simulink model "target_driver_2022_Ctrl_v_2_4_landing_2017a"  (R2017a)
settings: Solver=FixedStepDiscrete  StartTime=0.0  StopTime=13  FixedStep=0.0001  RelTol=1e-3  EnableMultiTasking=on
values from neighbouring files (symbols this model uses):
  a2_lb = -0.25    [target_driver_setup_2022_Ctrl_V_2_4.m]    (also in target_driver_setup_2022_Ctrl_V_2_4_christian.m)
  a2_openloop = -0    (= 0)    [target_driver_setup_2022_Ctrl_V_2_4.m]    (also in target_driver_setup_2022_Ctrl_V_2_4_christian.m)
  a2_ub = 0.25    [target_driver_setup_2022_Ctrl_V_2_4.m]    (also in target_driver_setup_2022_Ctrl_V_2_4_christian.m)
  adaptive_flag = 0    [target_driver_setup_2022_Ctrl_V_2_4.m]    (also in target_driver_setup_2022_Ctrl_V_2_4_christian.m)
  adaptive_gain = [gamma_adaptive, adaptive_roll_limit, adaptive_pitch_limit, adaptive_yaw_limit, c_2_adaptive, gamma_lateral_adaptive, adaptive_x_limit, adaptive_y_limit, adaptive_z_limit, c_1_adaptive]    [target_driver_setup_2022_Ctrl_V_2_4.m]    (also in target_driver_setup_2022_Ctrl_V_2_4_christian.m)
  adaptive_lateral_flag = 0    [target_driver_setup_2022_Ctrl_V_2_4.m]    (also in target_driver_setup_2022_Ctrl_V_2_4_christian.m)
  adaptive_pitch_init = 0    [target_driver_setup_2022_Ctrl_V_2_4.m]    (also in target_driver_setup_2022_Ctrl_V_2_4_christian.m)
  adaptive_pitch_limit = 0.1/(scale^2)    (= 1e-07)    [target_driver_setup_2022_Ctrl_V_2_4.m]    (also in target_driver_setup_2022_Ctrl_V_2_4_christian.m)
  adaptive_pitch_limit_low = -adaptive_pitch_limit    (= -1e-07)    [target_driver_setup_2022_Ctrl_V_2_4.m]    (also in target_driver_setup_2022_Ctrl_V_2_4_christian.m)
  adaptive_roll_init = 0    [target_driver_setup_2022_Ctrl_V_2_4.m]    (also in target_driver_setup_2022_Ctrl_V_2_4_christian.m)
  adaptive_roll_limit = 0.3/(scale^2)    (= 3e-07)    [target_driver_setup_2022_Ctrl_V_2_4.m]    (also in target_driver_setup_2022_Ctrl_V_2_4_christian.m)
  adaptive_roll_limit_low = -adaptive_roll_limit    (= -3e-07)    [target_driver_setup_2022_Ctrl_V_2_4.m]    (also in target_driver_setup_2022_Ctrl_V_2_4_christian.m)
  adaptive_x_init = 0    [target_driver_setup_2022_Ctrl_V_2_4.m]    (also in target_driver_setup_2022_Ctrl_V_2_4_christian.m)
  adaptive_x_limit = 0.15/(scale)    (= 0.00015)    [target_driver_setup_2022_Ctrl_V_2_4.m]    (also in target_driver_setup_2022_Ctrl_V_2_4_christian.m)
  adaptive_x_limit_low = -adaptive_x_limit    (= -0.00015)    [target_driver_setup_2022_Ctrl_V_2_4.m]    (also in target_driver_setup_2022_Ctrl_V_2_4_christian.m)
  adaptive_y_init = 0    [target_driver_setup_2022_Ctrl_V_2_4.m]    (also in target_driver_setup_2022_Ctrl_V_2_4_christian.m)
  adaptive_y_limit = 0.15/(scale)    (= 0.00015)    [target_driver_setup_2022_Ctrl_V_2_4.m]    (also in target_driver_setup_2022_Ctrl_V_2_4_christian.m)
  adaptive_y_limit_low = -adaptive_y_limit    (= -0.00015)    [target_driver_setup_2022_Ctrl_V_2_4.m]    (also in target_driver_setup_2022_Ctrl_V_2_4_christian.m)
  adaptive_yaw_init = 0    [target_driver_setup_2022_Ctrl_V_2_4.m]    (also in target_driver_setup_2022_Ctrl_V_2_4_christian.m)
  adaptive_yaw_limit = 0.035/(scale^2)    (= 3.5e-08)    [target_driver_setup_2022_Ctrl_V_2_4.m]    (also in target_driver_setup_2022_Ctrl_V_2_4_christian.m)
  adaptive_yaw_limit_low = -adaptive_yaw_limit    (= -3.5e-08)    [target_driver_setup_2022_Ctrl_V_2_4.m]    (also in target_driver_setup_2022_Ctrl_V_2_4_christian.m)
  adaptive_z_init = 0/scale    (= 0)    [target_driver_setup_2022_Ctrl_V_2_4.m]    (also in target_driver_setup_2022_Ctrl_V_2_4_christian.m)
  adaptive_z_limit = 0.20/(scale)    (= 0.0002)    [target_driver_setup_2022_Ctrl_V_2_4.m]    (also in target_driver_setup_2022_Ctrl_V_2_4_christian.m)
  adaptive_z_limit_low = -adaptive_z_limit/1    (= -0.0002)    [target_driver_setup_2022_Ctrl_V_2_4.m]    (also in target_driver_setup_2022_Ctrl_V_2_4_christian.m)
  att_s = 500    [target_driver_setup_2022_Ctrl_V_2_4.m]    (also in target_driver_setup_2022_Ctrl_V_2_4_christian.m)
  b_1_d_desired = [1,0,0]    [target_driver_setup_2022_Ctrl_V_2_4.m]    (also in target_driver_setup_2022_Ctrl_V_2_4_christian.m)
  closedloop_flag = 1    [target_driver_setup_2022_Ctrl_V_2_4.m]    (also in target_driver_setup_2022_Ctrl_V_2_4_christian.m)
  control_gain = [k_x,k_v, k_R, k_Omega, k_z, k_vz, k_Rx]    [target_driver_setup_2022_Ctrl_V_2_4.m]    (also in target_driver_setup_2022_Ctrl_V_2_4_christian.m)
  delay = delay-vicon_sample_cycle/2    [target_driver_setup_2022_Ctrl_V_2_4.m]    (also in target_driver_setup_2022_Ctrl_V_2_4_christian.m)
  drv_amp = 160    [target_driver_setup_2022_Ctrl_V_2_4.m]    (also in target_driver_setup_2022_Ctrl_V_2_4_christian.m)
  drv_bias = max_drv_bias    (= 300)    [target_driver_setup_2022_Ctrl_V_2_4.m]    (also in target_driver_setup_2022_Ctrl_V_2_4_christian.m)
  drv_pitch_left = 0    [target_driver_setup_2022_Ctrl_V_2_4.m]    (also in target_driver_setup_2022_Ctrl_V_2_4_christian.m)
  drv_pitch_right = 0    [target_driver_setup_2022_Ctrl_V_2_4.m]    (also in target_driver_setup_2022_Ctrl_V_2_4_christian.m)
  drv_roll = -2    [target_driver_setup_2022_Ctrl_V_2_4.m]    (also in target_driver_setup_2022_Ctrl_V_2_4_christian.m = 0)
  f_fin = f    (= 155)    [target_driver_setup_2022_Ctrl_V_2_4.m]    (also in target_driver_setup_2022_Ctrl_V_2_4_christian.m)
  f_int = f    (= 155)    [target_driver_setup_2022_Ctrl_V_2_4.m]    (also in target_driver_setup_2022_Ctrl_V_2_4_christian.m)
  g = 9.8    [target_driver_setup_2022_Ctrl_V_2_4.m]    (also in target_driver_setup_2022_Ctrl_V_2_4_christian.m)
  I_moment_vec = [Ixx, Iyy, Izz]    [target_driver_setup_2022_Ctrl_V_2_4.m]    (also in target_driver_setup_2022_Ctrl_V_2_4_christian.m)
  landing_flag = 0    [target_driver_setup_2022_Ctrl_V_2_4.m]    (also in target_driver_setup_2022_Ctrl_V_2_4_christian.m)
  landing_parameter = [start_delay+T,transition_rate, rising_time, falling_time, landing_rising_time, landing_z_decrease, landing_y_decrease, landing_x_decrease]    [target_driver_setup_2022_Ctrl_V_2_4.m]    (also in target_driver_setup_2022_Ctrl_V_2_4_christian.m = [start_delay+T, transition_rate, rising_time, falling_time, )
  low_bound = -8    [target_driver_setup_2022_Ctrl_V_2_4.m]    (also in target_driver_setup_2022_Ctrl_V_2_4_christian.m = -10)
  low_bound_eR = -0.8    [target_driver_setup_2022_Ctrl_V_2_4.m]    (also in target_driver_setup_2022_Ctrl_V_2_4_christian.m)
  low_bound_vx = -0.5    [target_driver_setup_2022_Ctrl_V_2_4.m]    (also in target_driver_setup_2022_Ctrl_V_2_4_christian.m)
  low_bound_vy = -0.5    [target_driver_setup_2022_Ctrl_V_2_4.m]    (also in target_driver_setup_2022_Ctrl_V_2_4_christian.m)
  low_bound_vz = -0.5    [target_driver_setup_2022_Ctrl_V_2_4.m]    (also in target_driver_setup_2022_Ctrl_V_2_4_christian.m)
  low_bound_x = -0.06    [target_driver_setup_2022_Ctrl_V_2_4.m]    (also in target_driver_setup_2022_Ctrl_V_2_4_christian.m)
  low_bound_y = -0.06    [target_driver_setup_2022_Ctrl_V_2_4.m]    (also in target_driver_setup_2022_Ctrl_V_2_4_christian.m)
  low_bound_z = -0.04    [target_driver_setup_2022_Ctrl_V_2_4.m]    (also in target_driver_setup_2022_Ctrl_V_2_4_christian.m)
  m = m+payload    (= 0.000124)    [target_driver_setup_2022_Ctrl_V_2_4.m]    (also in target_driver_setup_2022_Ctrl_V_2_4_christian.m = 0.000119)
  params_vec = [params_opt.delta_1, params_opt.delta_2, params_opt.delta_3, params_opt.gamma_1, params_opt.gamma_2, params_opt.gamma_3, params_opt.eta, params_opt.nu, params_opt.mu]'    [target_driver_setup_2022_Ctrl_V_2_4.m]    (also in target_driver_setup_2022_Ctrl_V_2_4_christian.m)
  phase = 0    [target_driver_setup_2022_Ctrl_V_2_4.m]    (also in target_driver_setup_2022_Ctrl_V_2_4_christian.m)
  r_desired = [default_x, default_y,z_desired]    [target_driver_setup_2022_Ctrl_V_2_4.m]    (also in target_driver_setup_2022_Ctrl_V_2_4_christian.m)
  roll_offset_angle = 0    [target_driver_setup_2022_Ctrl_V_2_4.m]    (also in target_driver_setup_2022_Ctrl_V_2_4_christian.m)
  running_time = start_delay+total_T    (= 8.5)    [target_driver_setup_2022_Ctrl_V_2_4.m]    (also in target_driver_setup_2022_Ctrl_V_2_4_christian.m = 8.4)
  running_time_control = start_delay_control+total_T+0.0    (= 8.6)    [target_driver_setup_2022_Ctrl_V_2_4.m]    (also in target_driver_setup_2022_Ctrl_V_2_4_christian.m = 8.5)
  start_delay = 2.0    (= 2)    [target_driver_setup_2022_Ctrl_V_2_4.m]    (also in target_driver_setup_2022_Ctrl_V_2_4_christian.m)
  start_delay_control = start_delay + ramp_delay    (= 2.1)    [target_driver_setup_2022_Ctrl_V_2_4.m]    (also in target_driver_setup_2022_Ctrl_V_2_4_christian.m)
  T = 0.5    [target_driver_setup_2022_Ctrl_V_2_4.m]    (also in target_driver_setup_2022_Ctrl_V_2_4_christian.m = 0.4)
  task_flag = 0    [target_driver_setup_2022_Ctrl_V_2_4.m]    (also in target_driver_setup_2022_Ctrl_V_2_4_christian.m)
  task_parameter = [radius_ref, frequency_ref, radius_ratio, lissajous_ratio, lissajous_delta, lissajous_amplitude_ratio,z_radius_ratio]    [target_driver_setup_2022_Ctrl_V_2_4.m]    (also in target_driver_setup_2022_Ctrl_V_2_4_christian.m)
  upp_bound = 8    [target_driver_setup_2022_Ctrl_V_2_4.m]    (also in target_driver_setup_2022_Ctrl_V_2_4_christian.m = 10)
  upp_bound_eR = 0.8    [target_driver_setup_2022_Ctrl_V_2_4.m]    (also in target_driver_setup_2022_Ctrl_V_2_4_christian.m)
  upp_bound_vx = 0.5    [target_driver_setup_2022_Ctrl_V_2_4.m]    (also in target_driver_setup_2022_Ctrl_V_2_4_christian.m)
  upp_bound_vy = 0.5    [target_driver_setup_2022_Ctrl_V_2_4.m]    (also in target_driver_setup_2022_Ctrl_V_2_4_christian.m)
  upp_bound_vz = 0.5    [target_driver_setup_2022_Ctrl_V_2_4.m]    (also in target_driver_setup_2022_Ctrl_V_2_4_christian.m)
  upp_bound_x = 0.06    [target_driver_setup_2022_Ctrl_V_2_4.m]    (also in target_driver_setup_2022_Ctrl_V_2_4_christian.m)
  upp_bound_y = 0.06    [target_driver_setup_2022_Ctrl_V_2_4.m]    (also in target_driver_setup_2022_Ctrl_V_2_4_christian.m)
  upp_bound_z = 0.04    [target_driver_setup_2022_Ctrl_V_2_4.m]    (also in target_driver_setup_2022_Ctrl_V_2_4_christian.m)
undefined symbols (not defined in the file or in its folder): A, Com1, DiscIntNeverNeededParam, left_mapping, left_mapping_F_to_Phi, lp_den, lp_num, none, right_mapping, right_mapping_F_to_Phi, vlp_den, vlp_num
libraries: simulink x25, xpcnilib x2, xpcseriallib x2, xpcutilitieslib x1
(part 1 of 4)
settings Model: ExtModeArmWhenConnect=off  Creator=DEAS IT  LastModifiedBy=Wyss User
settings SolverCC: EnableConcurrentExecution=on
settings DataIOCC: LimitDataPoints=on  MaxDataPoints=1000000000  SaveFormat=Array
settings OptimizationCC: BlockReduction=off  BooleanDataType=off  OptimizeBlockIOStorage=off  BufferReuse=off  GlobalBufferReuse=off  ExpressionFolding=off  ExpressionDepthLimit=2147483647  LocalBlockOutputs=off  InitFltsAndDblsToZero=on  OptimizeDataStoreBuffers=off  BusAssignmentInplaceUpdate=off
settings DebuggingCC: SaveWithParameterizedLinksMsg=none  UnderspecifiedInitializationDetection=Classic  MergeDetectMultiDrivingBlocksExec=none  MultiTaskDSMMsg=warning  MultiTaskCondExecSysMsg=none  FcnCallInpInsideContextMsg=warning  StateNameClashWarn=warning  SFUnexpectedBacktrackingDiag=warning  SFNoUnconditionalDefaultTransitionDiag=warning  SFExecutionAtInitializationDiag=none
settings HardwareCC: ProdBitPerPointer=32  ProdBitPerSizeT=32  ProdBitPerPtrDiffT=32  ProdLargestAtomicFloat=None  ProdWordSize=32  ProdLongLongMode=on  ProdHWDeviceType=Generic->32-bit x86 compatible  TargetHWDeviceType=32-bit Generic
settings ModelReferenceCC: PropagateSignalLabelsOutOfModel=off
settings RTWCC: SystemTargetFile=slrt.tlc  TemplateMakefile=slrt_default_tmf  Description=Simulink Real-Time  RTWCompilerOptimization=on
settings SimulinkRealTimeCC: TargetFcnLib=ansi_tfl_tmw.mat  RL32LogBufSizeModifier=10000000  xPCConcurrentTasks=on
settings ConfigComp: CovMetricSettings=dw  CovHtmlReporting=on  CovSaveCumulativeToWorkspaceVar=on  CovSaveSingleToWorkspaceVar=on  CovExternalEMLEnable=off

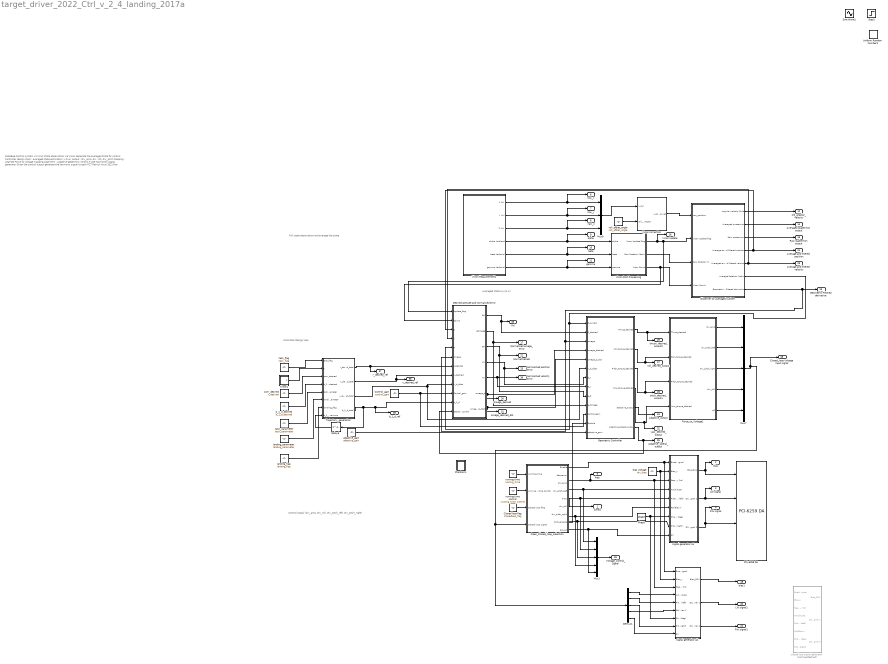
== system target_driver_2022_Ctrl_v_2_4_landing_2017a ==
  note: RoboBee Control system v2.1
      | Full state observation via Vicon
      | Generate the averaged state for control
      | Controller design
      | input : averaged state estimate (r,v,R,w)
      | output : drv_amp, drv_roll, drv_pitch
      | Mapping : Learned Force to voltage mapping
      | Algorithm : Adaptive geoemtric control T.Lee
      | Harmonitc signal generator
      | Given the control output generate the harmonic signal to each PZT
      |
      | Patrick Hyun 2021 Mar
  note: Controller Design loop
  note: Averaged state
      | (p,v,R,w)
  note: Full state observation and average the state
  note: Control signal
      | (drv_amp, drv_roll, drv_pitch_left, drv_pitch_right)
  Closed loop flag : Constant  Value=closedloop_flag
  Control_gain : Constant  Value=control_gain  SampleTime=-1
  Delay6 : Delay  DelayLength=1  InitialCondition=0
  Demux1 : Demux  Outputs=5
  Desired attitude and normalized error : Subsystem
  Force_to_Voltage1 : Subsystem
  Geometric Controller : Subsystem
  Mux1 : Mux  Inputs=5
  Mux7 : Mux  Inputs=5
  Mux9 : Mux  Inputs=3
  Observer for averaged system : Subsystem
  Open_Closed_loop_selection : Subsystem
  PCI-6259 DA : xpcnilib/D//A/M Series/PCI-6259 DA  channel=[1:4]  range=[10,5, 10, 10]  reset=[1 1 1 1]  initValue=[0 0 0 0]  sampletime=-1  slot=-1
      settings: SourceProductName=Simulink Real-Time  SourceProductBaseCode=XP
  Phantom1 : Subsystem
  Phase : Constant  Value=phase
  Trajectory_generation : MATLAB Function  TreatAsAtomicUnit=on
  Vicon Measurements : Subsystem
  Vicon Post Processing : Subsystem
  Vicon correction : MATLAB Function  TreatAsAtomicUnit=on
  adaptive_gain : Constant  Value=adaptive_gain  SampleTime=-1
  b_1_d_desired : Constant  Value=b_1_d_desired  SampleTime=-1
  bias voltage : Constant  Value=drv_bias
  closed loop signal generator : Subsystem  Commented=on
  com_desired : Constant  Value=r_desired  SampleTime=-1
  landing_flag : Constant  Value=landing_flag  SampleTime=-1
  landing_parameter : Constant  Value=landing_parameter  SampleTime=-1
  roll_offset_angle : Constant  Value=roll_offset_angle  SampleTime=-1
  running time : Constant  Value=running_time  SampleTime=-1
  running time control : Constant  Value=running_time_control  SampleTime=-1
  signal generator a1 : Subsystem
  signal generator a2 : Subsystem
  task_flag : Constant  Value=task_flag  SampleTime=-1
  task_parameter : Constant  Value=task_parameter  SampleTime=-1
  timer1 : Subsystem
  time1 : Outport
  bias : Outport  Port=2
  LW signal : Outport  Port=3
  RW signal : Outport  Port=4
  freq : Outport  Port=5
  raw_x : Outport  Port=6
  raw_y : Outport  Port=7
  raw_z : Outport  Port=8
  alpha : Outport  Port=9
  beta : Outport  Port=10
  gamma : Outport  Port=11
  "old_angular_velocity " : Outport  Port=12
  Geometric Filtered derivative : Outport  Port=13
  Averaged quaternion output : Outport  Port=14
  "Raw quaternion output " : Outport  Port=15
  Vicon Update : Outport  Port=16
  Normalized omega_error : Outport  Port=17
  Closed_loop Voltage input signal : Outport  Port=18
  bias1 : Outport  Port=19
  LW signal1 : Outport  Port=20
  RW signal1 : Outport  Port=21
  Normalized eR : Outport  Port=22
  Average and filtered velocity : Outport  Port=23
  "Average and filtered position " : Outport  Port=24
  Normalized position error : Outport  Port=25
  Voltage_control_Signal : Outport  Port=26
  roll_desired_output : Outport  Port=27
  pitch_desired_output1 : Outport  Port=28
  thrust_desired_output2 : Outport  Port=29
  omega_desired : Outport  Port=30
  omega_desired_dot : Outport  Port=31
  "yaw_desired_output " : Outport  Port=32
  Rd : Outport  Port=33
  Adaptive_output : Outport  Port=34
  Adaptive_lateral_output : Outport  Port=35
  Normalized velocity error : Outport  Port=36
  r_desired_ref : Outport  Port=37
  v_desired_ref : Outport  Port=38
  b_1_d_ref : Outport  Port=39
  Sine Wave1 : Sin  IOType=siggen  SampleTime=0
  Step1 : Step  IOType=siggen  SampleTime=0
  Uniform Random Number1 : UniformRandomNumber  IOType=siggen  SampleTime=0
  wires:
  signal generator a1/1(Bias_D2A) -> PCI-6259 DA/1, bias/1
  signal generator a1/2(D2A DriveSignal 1) -> LW signal/1, PCI-6259 DA/2
  signal generator a1/3(D2A DriveSignal 2) -> RW signal/1, PCI-6259 DA/3
  bias voltage/1 -> signal generator a2/2(Bias_v), signal generator a1/2(Bias_v)
  Phase/1 -> signal generator a2/7(Phase (deg)), signal generator a1/7(Phase (deg))
  Vicon Measurements/2(Y (m)) -> raw_y/1, Mux9/2
  Vicon Measurements/3(Z (m)) -> Mux9/3, raw_z/1
  Vicon Measurements/6(gamma (radians)) -> gamma/1, Vicon Post Processing/3(gamma)
  Vicon Measurements/5(beta (radians)) -> Vicon Post Processing/2(beta), beta/1
  Vicon Measurements/1(X (m)) -> raw_x/1, Mux9/1
  Vicon Measurements/4(alpha (radians)) -> Vicon Post Processing/1(alpha), alpha/1
  Mux7/1 -> Closed_loop Voltage input signal/1, Demux1/1, Open_Closed_loop_selection/4(Closed loop signal)
  signal generator a2/1(Bias_D2A) -> bias1/1
  signal generator a2/2(D2A DriveSignal 1) -> LW signal1/1
  signal generator a2/3(D2A DriveSignal 2) -> RW signal1/1
  Vicon Post Processing/1("Vicon Update Flag ") -> Vicon Update/1, Desired attitude and normalized error/1(Update_flag), Observer for averaged system/2(Vicon Update flag)
  Vicon Post Processing/2(Raw Rotation Matrix) -> Observer for averaged system/3("Raw Rotation M ")
  Vicon Post Processing/3("Vicon Count ") -> Desired attitude and normalized error/2(Count), Observer for averaged system/4(Vicon Count)
  Observer for averaged system/1("Angular velocity Euler ") -> "old_angular_velocity "/1
  Observer for averaged system/2(Averaged quaternion) -> Averaged quaternion output/1
  Observer for averaged system/3(Raw quaternion) -> "Raw quaternion output "/1
  Observer for averaged system/6(Average Rotation Matrix) -> Desired attitude and normalized error/5(R), Geometric Controller/1(R_current)
  Observer for averaged system/5(Averaged and filtered velocity) -> Average and filtered velocity/1, Desired attitude and normalized error/4(v)
  Observer for averaged system/4("Average and filtered position ") -> Desired attitude and normalized error/3(p), "Average and filtered position "/1
  Open_Closed_loop_selection/2(frequency) -> signal generator a2/3(frequency (hz)), signal generator a1/3(frequency (hz)), freq/1
  running time/1 -> Open_Closed_loop_selection/1(runnting time)
  running time control/1 -> Open_Closed_loop_selection/2("running time control ")
  Closed loop flag/1 -> Open_Closed_loop_selection/3(Closed loop flag)
  Open_Closed_loop_selection/3(drv_amp) -> signal generator a1/4(Amplitude), Mux1/1
  Open_Closed_loop_selection/4("drv_pitch_left ") -> signal generator a1/5(PitchBias V (left)), Mux1/2
  Open_Closed_loop_selection/5(time) -> time1/1
  Open_Closed_loop_selection/6("drv_roll ") -> signal generator a1/6(RollBias V), Mux1/4
  Open_Closed_loop_selection/7("drv_pitch_right ") -> signal generator a1/8(PitchBias V (right)), Mux1/3
  Demux1/1 -> signal generator a2/4(Amplitude)
  Demux1/2 -> signal generator a2/5(PitchBias V (left))
  Demux1/3 -> signal generator a2/8(PitchBias V (right))
  Demux1/4 -> signal generator a2/6(RollBias V)
  Mux1/1 -> Voltage_control_Signal/1
  Geometric Controller/3(Pitch_torque_desired) -> Force_to_Voltage1/3(Pitch_torque_desired), pitch_desired_output1/1
  Geometric Controller/1(Thrust_desired) -> thrust_desired_output2/1, Force_to_Voltage1/1("Thrust_desired ")
  Geometric Controller/2(roll_torque_desired) -> roll_desired_output/1, Force_to_Voltage1/2(Roll_torque_desired)
  Open_Closed_loop_selection/1("Enable ") -> signal generator a2/1(EnableSignal), signal generator a1/1(EnableSignal)
  Trajectory_generation/3(x_d_ddot_total) -> Desired attitude and normalized error/9(x_d_ddot), Geometric Controller/6(x_d_ddot)
  Control_gain/1 -> Geometric Controller/11(control_gain), Desired attitude and normalized error/10(Control_gain)
  Trajectory_generation/2(v_desired_total) -> v_desired_ref/1, Desired attitude and normalized error/8(v_desired)
  Desired attitude and normalized error/2(eOmega) -> Geometric Controller/10(e_Omega), Normalized omega_error/1
  Desired attitude and normalized error/3(eR) -> Geometric Controller/9(e_R), Normalized eR/1
  Desired attitude and normalized error/4(ex) -> Geometric Controller/7(e_x), Normalized position error/1
  Desired attitude and normalized error/1(Rd) -> Geometric Controller/2(R_desired), Rd/1
  Observer for averaged system/7(Geometric filtered derivative) -> Geometric Controller/3(omega), Desired attitude and normalized error/6(omega), Geometric Filtered derivative/1
  Desired attitude and normalized error/6(omega_d) -> Geometric Controller/4(omega_desired), omega_desired/1
  Desired attitude and normalized error/7(omega_d_ddot) -> Geometric Controller/5(omega_d_dot), omega_desired_dot/1
  Desired attitude and normalized error/5(ev) -> Normalized velocity error/1, Geometric Controller/8(e_v)
  Open_Closed_loop_selection/9(a2_out) -> Mux1/5, signal generator a1/9(a2)
  Open_Closed_loop_selection/8(Cntrl_enable) -> Geometric Controller/12(Enable)
  Geometric Controller/4(Yaw_torque_desired) -> "yaw_desired_output "/1, Force_to_Voltage1/4(Yaw_torque_desired)
  Force_to_Voltage1/1(drv_amp) -> Mux7/1
  Force_to_Voltage1/2(drv_pitch_left) -> Mux7/2
  Force_to_Voltage1/3(drv_pitch_right) -> Mux7/3
  Force_to_Voltage1/4(drv_roll) -> Mux7/4
  Force_to_Voltage1/5(a2) -> Mux7/5
  Demux1/5 -> signal generator a2/9(a2)
  Trajectory_generation/4(b_1_d_total) -> Delay6/1, b_1_d_ref/1, Desired attitude and normalized error/11(b_1_d)
  adaptive_gain/1 -> Geometric Controller/13(adaptive_gain)
  Geometric Controller/5(adaptive_output) -> Adaptive_output/1
  Geometric Controller/6(adaptive_lateral_output) -> Desired attitude and normalized error/12(adaptive_lateral_control), Adaptive_lateral_output/1
  Mux9/1 -> Vicon correction/1(x_cur)
  roll_offset_angle/1 -> Vicon correction/2(roll_offset_angle)
  Vicon correction/1(x_corrected_vec) -> Observer for averaged system/1("raw_position ")
  com_desired/1 -> Trajectory_generation/3(com_desired)
  Trajectory_generation/1(r_desired_total) -> r_desired_ref/1, Desired attitude and normalized error/7(r_desired)
  timer1/1(time) -> Trajectory_generation/2(t)
  task_flag/1 -> Trajectory_generation/1(task_flag)
  b_1_d_desired/1 -> Trajectory_generation/4(b_1_d_desired)
  task_parameter/1 -> Trajectory_generation/5(task_parameter)
  landing_parameter/1 -> Trajectory_generation/6(landing_parameter)
  landing_flag/1 -> Trajectory_generation/7(landing_flag)
  Delay6/1 -> Trajectory_generation/8(b_1_d_previous)

== system target_driver_2022_Ctrl_v_2_4_landing_2017a/Desired attitude and normalized error ==
  Update_flag : Inport
  Count : Inport  Port=2
  p : Inport  Port=3
  v : Inport  Port=4
  R : Inport  Port=5
  omega : Inport  Port=6
  r_desired : Inport  Port=7
  v_desired : Inport  Port=8
  x_d_ddot : Inport  Port=9
  Control_gain : Inport  Port=10
  b_1_d : Inport  Port=11
  adaptive_lateral_control : Inport  Port=12
  Delay6 : Delay  DelayLength=1  InitialCondition=0
  "Desired_Attitude " : MATLAB Function  TreatAsAtomicUnit=on
  Geometric derivative for Rd in SO(3) : Subsystem
  m : Constant  Value=m
  m1 : Constant  Value=g
  saturated normalized error observation : Subsystem
  Rd : Outport
  eOmega : Outport  Port=2
  eR : Outport  Port=3
  ex : Outport  Port=4
  ev : Outport  Port=5
  omega_d : Outport  Port=6
  omega_d_ddot : Outport  Port=7
  wires:
  r_desired/1 -> saturated normalized error observation/7(r_desired)
  x_d_ddot/1 -> "Desired_Attitude "/5(x_d_ddot)
  saturated normalized error observation/3("Normalized position error ") -> ex/1, "Desired_Attitude "/3(e_x)
  Delay6/1 -> Geometric derivative for Rd in SO(3)/1(Previous Averaged Rotation M), "Desired_Attitude "/2(R_d_prev)
  omega/1 -> saturated normalized error observation/4(omega)
  "Desired_Attitude "/1(R_d_vec) -> saturated normalized error observation/6(R_desired), Delay6/1, Rd/1, Geometric derivative for Rd in SO(3)/3(Current Averaged Rotation M)
  saturated normalized error observation/2(Normalized eR) -> eR/1
  Count/1 -> Geometric derivative for Rd in SO(3)/2(Vicon Count)
  Update_flag/1 -> "Desired_Attitude "/10(update), Geometric derivative for Rd in SO(3)/4("Vicon Update Flag ")
  p/1 -> saturated normalized error observation/1(p)
  Control_gain/1 -> "Desired_Attitude "/7(control_gain)
  v_desired/1 -> saturated normalized error observation/8("v_desired ")
  Geometric derivative for Rd in SO(3)/2(Filtered Geometric derivative ddRd in SO(3)1) -> omega_d_ddot/1
  v/1 -> saturated normalized error observation/2(v)
  saturated normalized error observation/1("Normalized omega error ") -> eOmega/1
  saturated normalized error observation/4(Normalized velocity error) -> "Desired_Attitude "/4(e_v), ev/1
  R/1 -> "Desired_Attitude "/1(R_cur), saturated normalized error observation/3(R)
  Geometric derivative for Rd in SO(3)/1(Filtered Geometric derivative dRd in SO(3)) -> saturated normalized error observation/5("omega_desired "), omega_d/1
  m/1 -> "Desired_Attitude "/8(m)
  m1/1 -> "Desired_Attitude "/9(g)
  b_1_d/1 -> "Desired_Attitude "/6(b_1_d)
  adaptive_lateral_control/1 -> "Desired_Attitude "/11(adaptive_lateral_control)

== system target_driver_2022_Ctrl_v_2_4_landing_2017a/Force_to_Voltage1 ==
  note: Mapping from desired Thrust/Torque to Wing traj to Voltage mapping
      |
      | Patrick Hyun 2021 Apr
  "Thrust_desired " : Inport
  Roll_torque_desired : Inport  Port=2
  Pitch_torque_desired : Inport  Port=3
  Yaw_torque_desired : Inport  Port=4
  A : Constant  Commented=on  Value=A
  Desired_Force_to_Voltage : MATLAB Function  TreatAsAtomicUnit=on
  "Force to Trajectory " : MATLAB Function  Commented=on  TreatAsAtomicUnit=on
  Saturation : Saturate  UpperLimit=a2_ub  LowerLimit=a2_lb
  "Trajectory to Voltage Input " : MATLAB Function  Commented=on  TreatAsAtomicUnit=on
  left_mapping : Constant  Commented=on  Value=left_mapping
  left_mapping_F_to_Phi : Constant  Commented=on  Value=left_mapping_F_to_Phi
  params_vec : Constant  Value=params_vec
  right_mapping1 : Constant  Commented=on  Value=right_mapping
  right_mapping_F_to_Phi : Constant  Commented=on  Value=right_mapping_F_to_Phi
  drv_amp : Outport
  drv_pitch_left : Outport  Port=2
  drv_pitch_right : Outport  Port=3
  drv_roll : Outport  Port=4
  a2 : Outport  Port=5
  wires:
  left_mapping/1 -> "Trajectory to Voltage Input "/4(left_mapping)
  right_mapping1/1 -> "Trajectory to Voltage Input "/5(right_mapping)
  A/1 -> "Force to Trajectory "/6(A)
  "Force to Trajectory "/1(Phi_left_p2p_desired) -> "Trajectory to Voltage Input "/1(Phi_left_p2p_command)
  "Force to Trajectory "/2(Phi_right_p2p_desired) -> "Trajectory to Voltage Input "/2(Phi_right_p2p_command)
  "Force to Trajectory "/3(Phi_pitch_desired) -> "Trajectory to Voltage Input "/3(Phi_pitch_command)
  left_mapping_F_to_Phi/1 -> "Force to Trajectory "/4(left_mapping_F_to_Phi)
  right_mapping_F_to_Phi/1 -> "Force to Trajectory "/5(right_mapping_F_to_Phi)
  Desired_Force_to_Voltage/4(drv_pitch_right) -> drv_pitch_right/1
  Desired_Force_to_Voltage/3(drv_pitch_left) -> drv_pitch_left/1
  Desired_Force_to_Voltage/2(drv_roll) -> drv_roll/1
  Desired_Force_to_Voltage/1(drv_amp) -> drv_amp/1
  "Thrust_desired "/1 -> Desired_Force_to_Voltage/1(Thrust_desired)
  Roll_torque_desired/1 -> Desired_Force_to_Voltage/2(Roll_torque_desired)
  Pitch_torque_desired/1 -> Desired_Force_to_Voltage/3(Pitch_torque_desired)
  Yaw_torque_desired/1 -> Desired_Force_to_Voltage/4(Yaw_torque_desired)
  params_vec/1 -> Desired_Force_to_Voltage/5(params_vec)
  Desired_Force_to_Voltage/5(a2_coeff) -> Saturation/1
  Saturation/1 -> a2/1

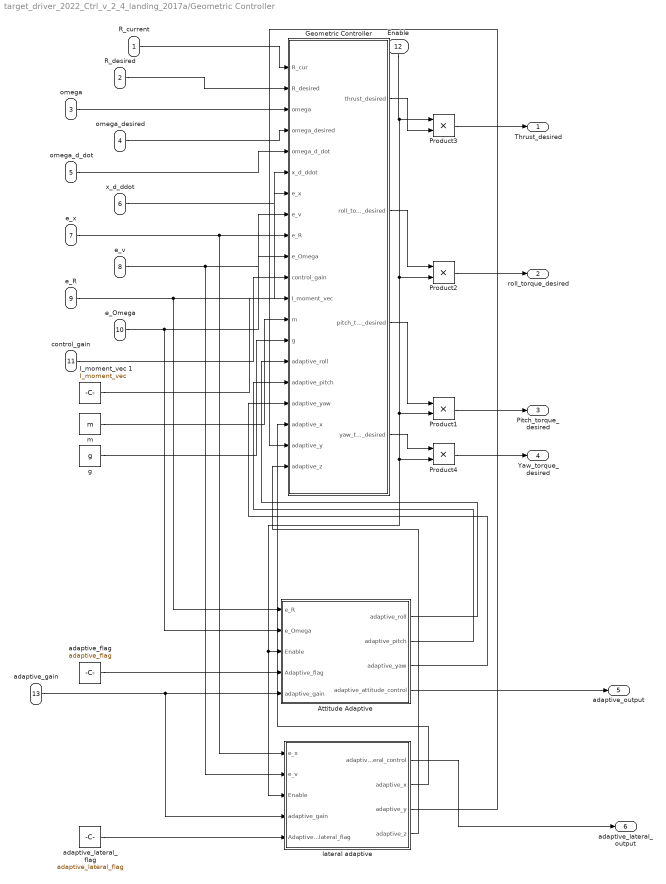
== system target_driver_2022_Ctrl_v_2_4_landing_2017a/Geometric Controller ==
  R_current : Inport
  R_desired : Inport  Port=2
  omega : Inport  Port=3
  omega_desired : Inport  Port=4
  omega_d_dot : Inport  Port=5
  x_d_ddot : Inport  Port=6
  e_x : Inport  Port=7
  e_v : Inport  Port=8
  e_R : Inport  Port=9
  e_Omega : Inport  Port=10
  control_gain : Inport  Port=11
  Enable : Inport  Port=12
  adaptive_gain : Inport  Port=13
  Attitude Adaptive : Subsystem
  Geometric Controller : MATLAB Function  TreatAsAtomicUnit=on
  I_moment_vec 1 : Constant  Value=I_moment_vec
  Product{1..4} (4 alike) : Product  RndMeth=Zero
  adaptive_flag : Constant  Value=adaptive_flag
  adaptive_lateral_flag : Constant  Value=adaptive_lateral_flag
  g : Constant  Value=g
  lateral adaptive : Subsystem
  m : Constant  Value=m
  Thrust_desired : Outport
  roll_torque_desired : Outport  Port=2
  Pitch_torque_desired : Outport  Port=3
  Yaw_torque_desired : Outport  Port=4
  adaptive_output : Outport  Port=5
  adaptive_lateral_output : Outport  Port=6
  wires:
  Product3/1 -> Thrust_desired/1
  Geometric Controller/3(pitch_torque_desired) -> Product1/1
  I_moment_vec 1/1 -> Geometric Controller/12(I_moment_vec)
  Product2/1 -> roll_torque_desired/1
  Product1/1 -> Pitch_torque_desired/1
  Geometric Controller/2(roll_torque_desired) -> Product2/1
  R_current/1 -> Geometric Controller/1(R_cur)
  Geometric Controller/1(thrust_desired) -> Product3/2
  R_desired/1 -> Geometric Controller/2(R_desired)
  omega/1 -> Geometric Controller/3(omega)
  omega_desired/1 -> Geometric Controller/4(omega_desired)
  omega_d_dot/1 -> Geometric Controller/5(omega_d_dot)
  e_R/1 -> Attitude Adaptive/1(e_R), Geometric Controller/9(e_R)
  e_Omega/1 -> Attitude Adaptive/2(e_Omega), Geometric Controller/10(e_Omega)
  control_gain/1 -> Geometric Controller/11(control_gain)
  g/1 -> Geometric Controller/14(g)
  m/1 -> Geometric Controller/13(m)
  x_d_ddot/1 -> Geometric Controller/6(x_d_ddot)
  adaptive_flag/1 -> Attitude Adaptive/4(Adaptive_flag)
  adaptive_gain/1 -> lateral adaptive/4(adaptive_gain), Attitude Adaptive/5(adaptive_gain)
  Attitude Adaptive/1(adaptive_roll) -> Geometric Controller/15(adaptive_roll)
  Attitude Adaptive/2(adaptive_pitch) -> Geometric Controller/16(adaptive_pitch)
  Attitude Adaptive/3(adaptive_yaw) -> Geometric Controller/17(adaptive_yaw)
  Attitude Adaptive/4(adaptive_attitude_control) -> adaptive_output/1
  Enable/1 -> Product4/2, Attitude Adaptive/3(Enable), lateral adaptive/3(Enable), Product1/2, Product2/2, Product3/1
  Geometric Controller/4(yaw_torque_desired) -> Product4/1
  Product4/1 -> Yaw_torque_desired/1
  e_x/1 -> Geometric Controller/7(e_x), lateral adaptive/1(e_x)
  e_v/1 -> lateral adaptive/2(e_v), Geometric Controller/8(e_v)
  adaptive_lateral_flag/1 -> lateral adaptive/5(Adaptive_lateral_flag)
  lateral adaptive/1(adaptive_lateral_control) -> adaptive_lateral_output/1
  lateral adaptive/2(adaptive_x) -> Geometric Controller/18(adaptive_x)
  lateral adaptive/3(adaptive_y) -> Geometric Controller/19(adaptive_y)
  lateral adaptive/4(adaptive_z) -> Geometric Controller/20(adaptive_z)

== system target_driver_2022_Ctrl_v_2_4_landing_2017a/Observer for averaged system ==
  note: Observer for averaged system using geoemtric average
      | Includes the Euler derivatives to compute the angular velocity (probably not used for control)
      | Includes the geometric average and the first order derivative in Riemannian metric SO(3)
      |
      | Patrick 2021 Mar
  "raw_position " : Inport
  Vicon Update flag : Inport  Port=2
  "Raw Rotation M " : Inport  Port=3
  Vicon Count : Inport  Port=4
  Attitude Observer : Subsystem
  "Euler derivative & filtered angular velocity " : Subsystem
  Position Observer : Subsystem
  Terminator : Terminator
  "Angular velocity Euler " : Outport
  Averaged quaternion : Outport  Port=2
  Raw quaternion : Outport  Port=3
  "Average and filtered position " : Outport  Port=4
  Averaged and filtered velocity : Outport  Port=5
  Average Rotation Matrix : Outport  Port=6
  Geometric filtered derivative : Outport  Port=7
  wires:
  "Raw Rotation M "/1 -> "Euler derivative & filtered angular velocity "/1("Rotation matrix "), Attitude Observer/2(Raw Rotation)
  Vicon Count/1 -> Attitude Observer/3(Vicon Count), Position Observer/3(Vicon Count)
  "raw_position "/1 -> Position Observer/1("raw_position ")
  Position Observer/1(Average and filtered position) -> "Average and filtered position "/1
  Position Observer/2(Averaged and filtered velocity) -> Averaged and filtered velocity/1
  "Euler derivative & filtered angular velocity "/1(Angular velocity_Euler) -> "Angular velocity Euler "/1
  Vicon Update flag/1 -> Attitude Observer/1(Vicon Update flag), Position Observer/2(vicon Update)
  Attitude Observer/1("Averaged quaternion ") -> Averaged quaternion/1
  Attitude Observer/2(Average Rotation Matrix) -> Average Rotation Matrix/1
  Attitude Observer/3(Raw quaternion) -> Raw quaternion/1
  Attitude Observer/4(Geometric filtered derivative) -> Geometric filtered derivative/1
  "Euler derivative & filtered angular velocity "/2(Frob_norm error) -> Terminator/1

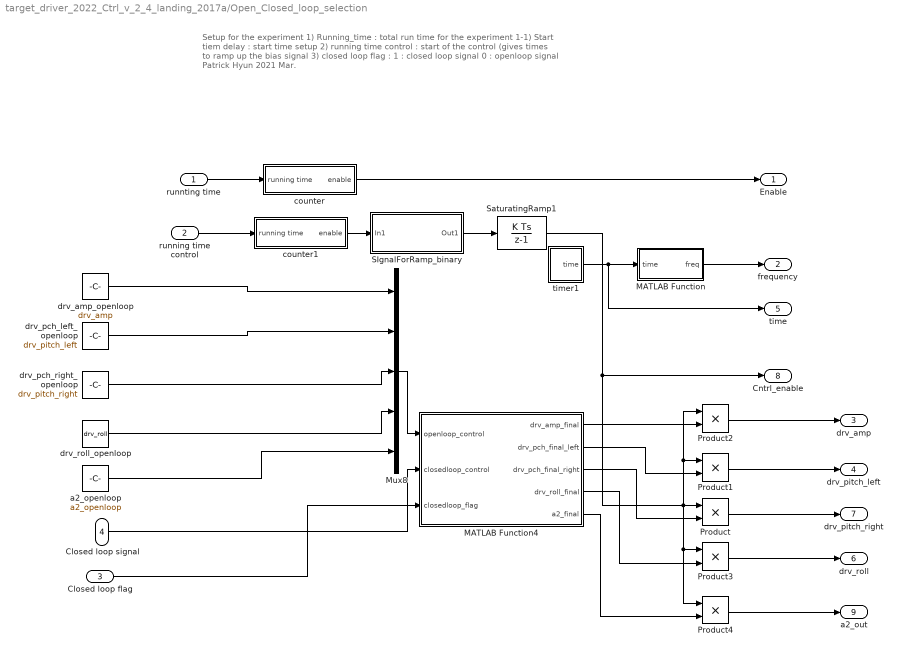
== system target_driver_2022_Ctrl_v_2_4_landing_2017a/Open_Closed_loop_selection ==
  note: Setup for the experiment
      |
      | 1) Running_time : total run time for the experiment
      | 1-1) Start tiem delay : start time setup
      | 2) running time control : start of the control (gives times to ramp up the bias signal
      | 3) closed loop flag : 1 : closed loop signal 0 : openloop signal
      |
      | Patrick Hyun 2021 Mar.
  runnting time : Inport
  "running time control " : Inport  Port=2
  Closed loop flag : Inport  Port=3
  Closed loop signal : Inport  Port=4
  MATLAB Function : MATLAB Function  TreatAsAtomicUnit=on
  MATLAB Function4 : MATLAB Function  TreatAsAtomicUnit=on
  Mux8 : Mux  Inputs=5
  Product{,1..4} (5 alike) : Product  RndMeth=Zero
  SIgnalForRamp_binary : Subsystem
  SaturatingRamp1 : DiscreteIntegrator  gainval=10  SampleTime=-1  LimitOutput=on  UpperSaturationLimit=1  LowerSaturationLimit=0  ICPrevOutput=DiscIntNeverNeededParam  ICPrevScaledInput=DiscIntNeverNeededParam
  a2_openloop : Constant  Value=a2_openloop
  counter : Subsystem
  counter1 : Subsystem
  "drv_amp_openloop " : Constant  Value=drv_amp
  drv_pch_left_openloop : Constant  Value=drv_pitch_left
  drv_pch_right_openloop : Constant  Value=drv_pitch_right
  "drv_roll_openloop " : Constant  Value=drv_roll
  timer1 : Subsystem
  "Enable " : Outport
  frequency : Outport  Port=2
  drv_amp : Outport  Port=3
  "drv_pitch_left " : Outport  Port=4
  time : Outport  Port=5
  "drv_roll " : Outport  Port=6
  "drv_pitch_right " : Outport  Port=7
  Cntrl_enable : Outport  Port=8
  a2_out : Outport  Port=9
  wires:
  runnting time/1 -> counter/1(running time)
  timer1/1(time) -> time/1, MATLAB Function/1(time)
  MATLAB Function/1(freq) -> frequency/1
  SIgnalForRamp_binary/1(Out1) -> SaturatingRamp1/1
  "drv_amp_openloop "/1 -> Mux8/1
  Product1/1 -> "drv_pitch_left "/1
  counter1/1(enable) -> SIgnalForRamp_binary/1(In1)
  "running time control "/1 -> counter1/1(running time)
  Product3/1 -> "drv_roll "/1
  SaturatingRamp1/1 -> Cntrl_enable/1, Product4/1, Product3/1, Product2/1, Product1/1, Product/1
  Closed loop flag/1 -> MATLAB Function4/3(closedloop_flag)
  MATLAB Function4/4(drv_roll_final) -> Product3/2
  Mux8/1 -> MATLAB Function4/1(openloop_control)
  MATLAB Function4/2(drv_pch_final_left) -> Product1/2
  Product2/1 -> drv_amp/1
  MATLAB Function4/1(drv_amp_final) -> Product2/2
  drv_pch_left_openloop/1 -> Mux8/2
  MATLAB Function4/3(drv_pch_final_right) -> Product/2
  Product/1 -> "drv_pitch_right "/1
  counter/1(enable) -> "Enable "/1
  Closed loop signal/1 -> MATLAB Function4/2(closedloop_control)
  "drv_roll_openloop "/1 -> Mux8/4
  drv_pch_right_openloop/1 -> Mux8/3
  Product4/1 -> a2_out/1
  MATLAB Function4/5(a2_final) -> Product4/2
  a2_openloop/1 -> Mux8/5

== system target_driver_2022_Ctrl_v_2_4_landing_2017a/Phantom1 ==
  note: high-speed camera trigger
  PCI-6259 DO1 : xpcnilib/Digital Output/M Series/PCI-6259 DO  channel=[1 2]  reset=[0 0]  initValue=[0 0]  sampletime=0.0001  slot=-1
      settings: SourceProductName=Simulink Real-Time  SourceProductBaseCode=XP
  Switch2 : Switch  Criteria=u2 > Threshold
  conv : DataTypeConversion  OutDataTypeStr=double
  pretrigger : Constant
  start at three : MATLAB Function  TreatAsAtomicUnit=on
  timer1 : Subsystem
  trigger_camera : Constant
  zero : Constant  Value=0
  wires:
  timer1/1(time) -> start at three/1(time)
  start at three/1(trigger) -> Switch2/1
  Switch2/1 -> conv/1
  zero/1 -> Switch2/3
  trigger_camera/1 -> Switch2/2
  conv/1 -> PCI-6259 DO1/2
  pretrigger/1 -> PCI-6259 DO1/1

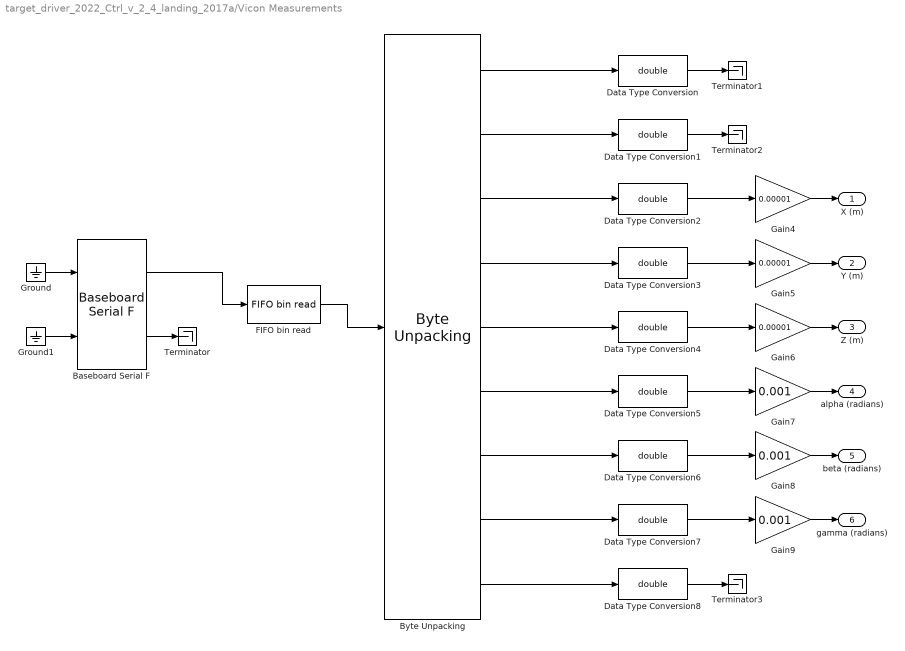
== system target_driver_2022_Ctrl_v_2_4_landing_2017a/Vicon Measurements ==
  Baseboard Serial F : xpcseriallib/Mainboard/Baseboard Serial F  group=FIFO Setup  port=1  irqnum=4  saddr1=0x3f8  saddr2=0x3e8  config=Com1/none  baud1=115200  parity1=None  ndata1=8  nstop1=1  fifomode1=16 deep  rlevel1=half full  automode1=on  xmtfifosize1=1024  xmtdatatype1=8 bit int null terminated  rcvfifosize1=1024  baud2=115200  parity2=None  ndata2=8  nstop2=1  fifomode2=16 deep  rlevel2=half full  automode2=off  xmtfifosize2=1024  xmtdatatype2=8 bit uint null terminated  rcvfifosize2=1024
      settings: SourceProductName=Simulink Real-Time  SourceProductBaseCode=XP
  "Byte Unpacking " : xpcutilitieslib/Byte Unpacking   MaskUnpackedDataTypes={'uint8','int16','int16','int16','int16','int16','int16','int16','uint8'}  MaskUnpackedDataSizes={[1] [1] [1] [1] [1] [1] [1] [1] [1]}  MaskAlignment=1
      settings: SourceProductName=Simulink Real-Time  SourceProductBaseCode=XP
  Data Type Conversion{,1..8} (9 alike) : DataTypeConversion  OutDataTypeStr=double
  "FIFO bin read " : xpcseriallib/FIFO bin read   header=[128,127,127]  lengths=[15]  hold=Hold last output if no new data  enable=off  maxsize=15  outputtype=8 bit uint null terminated  sampletime=0.0001
      settings: SourceProductName=Simulink Real-Time  SourceProductBaseCode=XP
  Gain4 : Gain  Gain=0.00001
  Gain5 : Gain  Gain=0.00001
  Gain6 : Gain  Gain=0.00001
  Gain7 : Gain  Gain=0.001
  Gain8 : Gain  Gain=0.001
  Gain9 : Gain  Gain=0.001
  Ground : Ground
  Ground1 : Ground
  Terminator{,1..3} (4 alike) : Terminator
  X (m) : Outport
  Y (m) : Outport  Port=2
  Z (m) : Outport  Port=3
  alpha (radians) : Outport  Port=4
  beta (radians) : Outport  Port=5
  gamma (radians) : Outport  Port=6
  wires:
  Baseboard Serial F/1 -> "FIFO bin read "/1
  Baseboard Serial F/2 -> Terminator/1
  Ground1/1 -> Baseboard Serial F/2
  Ground/1 -> Baseboard Serial F/1
  "Byte Unpacking "/1 -> Data Type Conversion/1
  "Byte Unpacking "/2 -> Data Type Conversion1/1
  "Byte Unpacking "/3 -> Data Type Conversion2/1
  "Byte Unpacking "/4 -> Data Type Conversion3/1
  "FIFO bin read "/1 -> "Byte Unpacking "/1
  "Byte Unpacking "/8 -> Data Type Conversion7/1
  "Byte Unpacking "/7 -> Data Type Conversion6/1
  "Byte Unpacking "/5 -> Data Type Conversion4/1
  "Byte Unpacking "/6 -> Data Type Conversion5/1
  Data Type Conversion3/1 -> Gain5/1
  Data Type Conversion4/1 -> Gain6/1
  Data Type Conversion5/1 -> Gain7/1
  Data Type Conversion6/1 -> Gain8/1
  Data Type Conversion7/1 -> Gain9/1
  "Byte Unpacking "/9 -> Data Type Conversion8/1
  Gain4/1 -> X (m)/1
  Data Type Conversion2/1 -> Gain4/1
  Gain5/1 -> Y (m)/1
  Gain6/1 -> Z (m)/1
  Gain7/1 -> alpha (radians)/1
  Gain8/1 -> beta (radians)/1
  Gain9/1 -> gamma (radians)/1
  Data Type Conversion/1 -> Terminator1/1
  Data Type Conversion1/1 -> Terminator2/1
  Data Type Conversion8/1 -> Terminator3/1

== system target_driver_2022_Ctrl_v_2_4_landing_2017a/Vicon Post Processing ==
  note: Process Vicon data
      |
      | 1) Generate Raw rotation matrix
      | 2) Flag the update of new vicon data
      | 3) Count the number of samples before new update
      |
      | By Patrick 2021 Mar
  alpha : Inport
  beta : Inport  Port=2
  gamma : Inport  Port=3
  Raw rotation matrix : Subsystem
  Vicon Validity check : Subsystem
  Vicon correction : MATLAB Function  TreatAsAtomicUnit=on
  roll_offset_angle : Constant  Value=roll_offset_angle  SampleTime=-1
  "Vicon Update Flag " : Outport
  Raw Rotation Matrix : Outport  Port=2
  "Vicon Count " : Outport  Port=3
  wires:
  Vicon Validity check/2(Vicon Count) -> "Vicon Count "/1
  beta/1 -> Raw rotation matrix/2(beta)
  gamma/1 -> Raw rotation matrix/3(gamma)
  alpha/1 -> Raw rotation matrix/1(alpha)
  Vicon Validity check/1("Vicon Update flag ") -> "Vicon Update Flag "/1
  roll_offset_angle/1 -> Vicon correction/2(roll_offset_angle)
  Raw rotation matrix/1(R) -> Vicon correction/1(R_cur)
  Vicon correction/1(Rot_corrected_vec) -> Raw Rotation Matrix/1, Vicon Validity check/1("Rotation Matrix ")

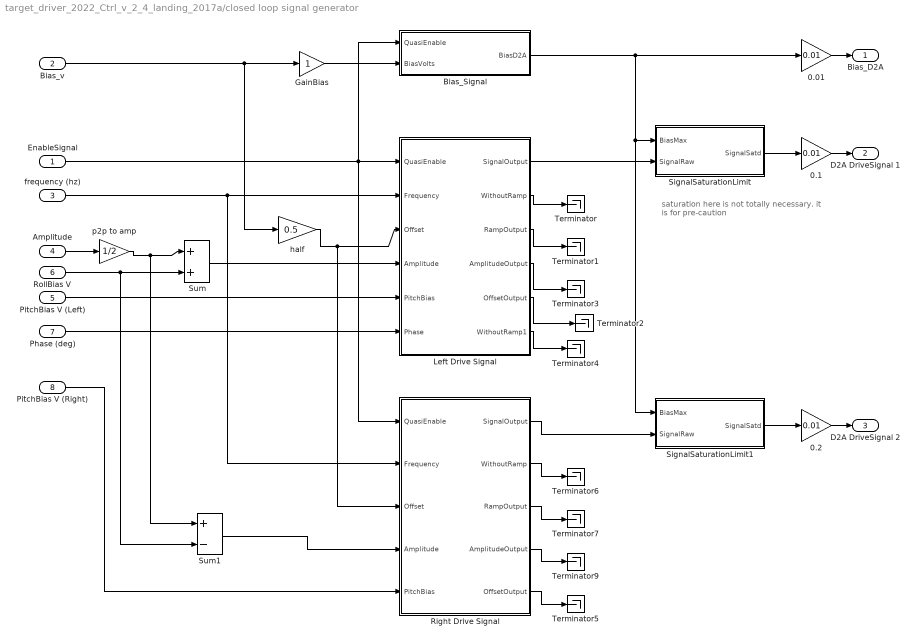
== system target_driver_2022_Ctrl_v_2_4_landing_2017a/closed loop signal generator ==
  note: saturation here is not totally necessary.
      | it is for pre-caution
  EnableSignal : Inport
  Bias_v : Inport  Port=2
  frequency (hz) : Inport  Port=3
  Amplitude : Inport  Port=4
  PitchBias V (Left) : Inport  Port=5
  RollBias V : Inport  Port=6
  Phase (deg) : Inport  Port=7
  PitchBias V (Right) : Inport  Port=8
  0.01 : Gain  Gain=0.01
  0.1 : Gain  Gain=0.01
  0.2 : Gain  Gain=0.01
  Bias_Signal : Subsystem
  GainBias : Gain
  "Left Drive Signal " : Subsystem
  Right Drive Signal : Subsystem
  SignalSaturationLimit : Subsystem
  SignalSaturationLimit1 : Subsystem
  Sum : Sum
  Sum1 : Sum  Inputs=+-
  Terminator{,1..7,9} (9 alike) : Terminator
  half : Gain  Gain=0.5
  p2p to amp : Gain  Gain=1/2
  Bias_D2A : Outport
  D2A DriveSignal 1 : Outport  Port=2
  D2A DriveSignal 2 : Outport  Port=3
  wires:
  Bias_Signal/1(BiasD2A) -> SignalSaturationLimit1/1(BiasMax), SignalSaturationLimit/1(BiasMax), 0.01/1
  half/1 -> "Left Drive Signal "/3(Offset), Right Drive Signal/3(Offset)
  Bias_v/1 -> GainBias/1, half/1
  EnableSignal/1 -> "Left Drive Signal "/1(QuasiEnable), Bias_Signal/1(QuasiEnable), Right Drive Signal/1(QuasiEnable)
  frequency (hz)/1 -> Right Drive Signal/2(Frequency), "Left Drive Signal "/2(Frequency)
  "Left Drive Signal "/2(WithoutRamp) -> Terminator/1
  "Left Drive Signal "/3(RampOutput) -> Terminator1/1
  "Left Drive Signal "/5(OffsetOutput) -> Terminator2/1
  SignalSaturationLimit/1(SignalSatd) -> 0.1/1
  GainBias/1 -> Bias_Signal/2(BiasVolts)
  Sum/1 -> "Left Drive Signal "/4(Amplitude)
  RollBias V/1 -> Sum/2, Sum1/2
  SignalSaturationLimit1/1(SignalSatd) -> 0.2/1
  Right Drive Signal/5(OffsetOutput) -> Terminator5/1
  Amplitude/1 -> p2p to amp/1
  p2p to amp/1 -> Sum/1, Sum1/1
  "Left Drive Signal "/4(AmplitudeOutput) -> Terminator3/1
  Right Drive Signal/2(WithoutRamp) -> Terminator6/1
  Right Drive Signal/3(RampOutput) -> Terminator7/1
  Right Drive Signal/4(AmplitudeOutput) -> Terminator9/1
  0.01/1 -> Bias_D2A/1
  0.1/1 -> D2A DriveSignal 1/1
  0.2/1 -> D2A DriveSignal 2/1
  Sum1/1 -> Right Drive Signal/4(Amplitude)
  Right Drive Signal/1(SignalOutput) -> SignalSaturationLimit1/2(SignalRaw)
  "Left Drive Signal "/1(SignalOutput) -> SignalSaturationLimit/2(SignalRaw)
  Phase (deg)/1 -> "Left Drive Signal "/6(Phase)
  "Left Drive Signal "/6(WithoutRamp1) -> Terminator4/1
  PitchBias V (Left)/1 -> "Left Drive Signal "/5(PitchBias)
  PitchBias V (Right)/1 -> Right Drive Signal/5(PitchBias)

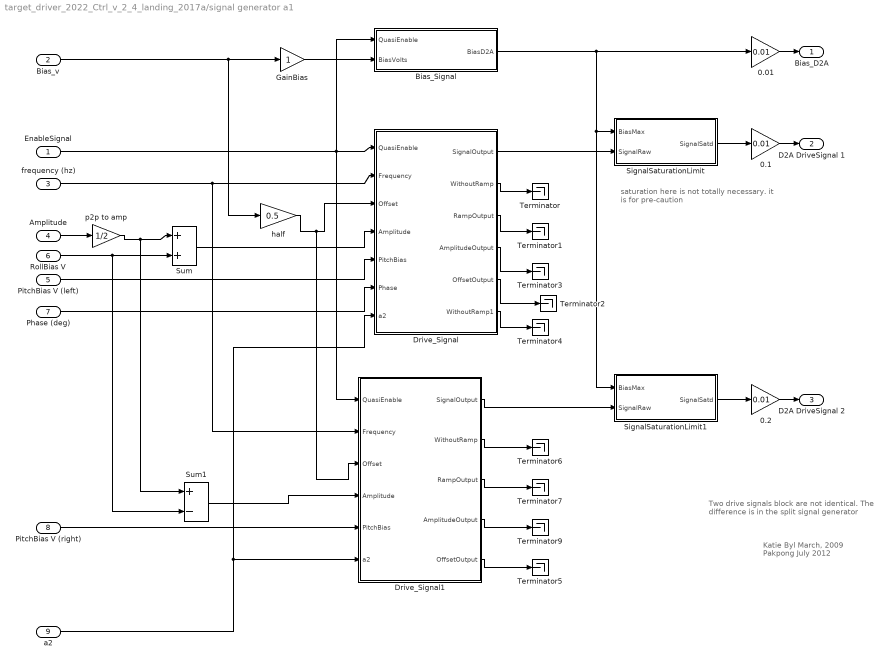
== system target_driver_2022_Ctrl_v_2_4_landing_2017a/signal generator a1 ==
  note: Katie Byl
      | March, 2009
      |
      | Pakpong
      | July 2012
  note: Two drive signals block are not identical.
      | The difference is in the split signal generator
  note: saturation here is not totally necessary.
      | it is for pre-caution
  EnableSignal : Inport
  Bias_v : Inport  Port=2
  frequency (hz) : Inport  Port=3
  Amplitude : Inport  Port=4
  PitchBias V (left) : Inport  Port=5
  RollBias V : Inport  Port=6
  Phase (deg) : Inport  Port=7
  PitchBias V (right) : Inport  Port=8
  a2 : Inport  Port=9
  0.01 : Gain  Gain=0.01
  0.1 : Gain  Gain=0.01
  0.2 : Gain  Gain=0.01
  Bias_Signal : Subsystem
  Drive_Signal : Subsystem
  Drive_Signal1 : Subsystem
  GainBias : Gain
  SignalSaturationLimit : Subsystem
  SignalSaturationLimit1 : Subsystem
  Sum : Sum
  Sum1 : Sum  Inputs=+-
  Terminator{,1..7,9} (9 alike) : Terminator
  half : Gain  Gain=0.5
  p2p to amp : Gain  Gain=1/2
  Bias_D2A : Outport
  D2A DriveSignal 1 : Outport  Port=2
  D2A DriveSignal 2 : Outport  Port=3
  wires:
  Bias_Signal/1(BiasD2A) -> SignalSaturationLimit1/1(BiasMax), SignalSaturationLimit/1(BiasMax), 0.01/1
  half/1 -> Drive_Signal/3(Offset), Drive_Signal1/3(Offset)
  Bias_v/1 -> GainBias/1, half/1
  EnableSignal/1 -> Drive_Signal/1(QuasiEnable), Bias_Signal/1(QuasiEnable), Drive_Signal1/1(QuasiEnable)
  frequency (hz)/1 -> Drive_Signal1/2(Frequency), Drive_Signal/2(Frequency)
  Drive_Signal/2(WithoutRamp) -> Terminator/1
  Drive_Signal/3(RampOutput) -> Terminator1/1
  Drive_Signal/5(OffsetOutput) -> Terminator2/1
  SignalSaturationLimit/1(SignalSatd) -> 0.1/1
  GainBias/1 -> Bias_Signal/2(BiasVolts)
  Sum/1 -> Drive_Signal/4(Amplitude)
  RollBias V/1 -> Sum/2, Sum1/2
  SignalSaturationLimit1/1(SignalSatd) -> 0.2/1
  Drive_Signal1/5(OffsetOutput) -> Terminator5/1
  Amplitude/1 -> p2p to amp/1
  p2p to amp/1 -> Sum/1, Sum1/1
  Drive_Signal/4(AmplitudeOutput) -> Terminator3/1
  Drive_Signal1/2(WithoutRamp) -> Terminator6/1
  Drive_Signal1/3(RampOutput) -> Terminator7/1
  Drive_Signal1/4(AmplitudeOutput) -> Terminator9/1
  0.01/1 -> Bias_D2A/1
  0.1/1 -> D2A DriveSignal 1/1
  0.2/1 -> D2A DriveSignal 2/1
  Sum1/1 -> Drive_Signal1/4(Amplitude)
  Drive_Signal1/1(SignalOutput) -> SignalSaturationLimit1/2(SignalRaw)
  Drive_Signal/1(SignalOutput) -> SignalSaturationLimit/2(SignalRaw)
  Phase (deg)/1 -> Drive_Signal/6(Phase)
  Drive_Signal/6(WithoutRamp1) -> Terminator4/1
  PitchBias V (left)/1 -> Drive_Signal/5(PitchBias)
  a2/1 -> Drive_Signal/7("a2 "), Drive_Signal1/6(a2)
  PitchBias V (right)/1 -> Drive_Signal1/5(PitchBias)

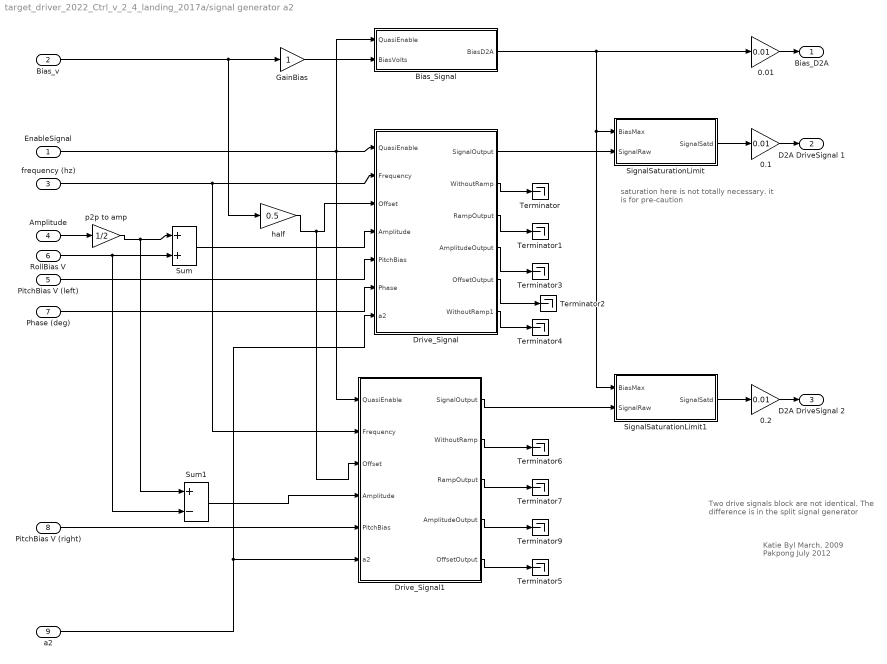
== system target_driver_2022_Ctrl_v_2_4_landing_2017a/signal generator a2 ==
  note: Katie Byl
      | March, 2009
      |
      | Pakpong
      | July 2012
  note: Two drive signals block are not identical.
      | The difference is in the split signal generator
  note: saturation here is not totally necessary.
      | it is for pre-caution
  EnableSignal : Inport
  Bias_v : Inport  Port=2
  frequency (hz) : Inport  Port=3
  Amplitude : Inport  Port=4
  PitchBias V (left) : Inport  Port=5
  RollBias V : Inport  Port=6
  Phase (deg) : Inport  Port=7
  PitchBias V (right) : Inport  Port=8
  a2 : Inport  Port=9
  0.01 : Gain  Gain=0.01
  0.1 : Gain  Gain=0.01
  0.2 : Gain  Gain=0.01
  Bias_Signal : Subsystem
  Drive_Signal : Subsystem
  Drive_Signal1 : Subsystem
  GainBias : Gain
  SignalSaturationLimit : Subsystem
  SignalSaturationLimit1 : Subsystem
  Sum : Sum
  Sum1 : Sum  Inputs=+-
  Terminator{,1..7,9} (9 alike) : Terminator
  half : Gain  Gain=0.5
  p2p to amp : Gain  Gain=1/2
  Bias_D2A : Outport
  D2A DriveSignal 1 : Outport  Port=2
  D2A DriveSignal 2 : Outport  Port=3
  wires:
  Bias_Signal/1(BiasD2A) -> SignalSaturationLimit1/1(BiasMax), SignalSaturationLimit/1(BiasMax), 0.01/1
  half/1 -> Drive_Signal/3(Offset), Drive_Signal1/3(Offset)
  Bias_v/1 -> GainBias/1, half/1
  EnableSignal/1 -> Drive_Signal/1(QuasiEnable), Bias_Signal/1(QuasiEnable), Drive_Signal1/1(QuasiEnable)
  frequency (hz)/1 -> Drive_Signal1/2(Frequency), Drive_Signal/2(Frequency)
  Drive_Signal/2(WithoutRamp) -> Terminator/1
  Drive_Signal/3(RampOutput) -> Terminator1/1
  Drive_Signal/5(OffsetOutput) -> Terminator2/1
  SignalSaturationLimit/1(SignalSatd) -> 0.1/1
  GainBias/1 -> Bias_Signal/2(BiasVolts)
  Sum/1 -> Drive_Signal/4(Amplitude)
  RollBias V/1 -> Sum/2, Sum1/2
  SignalSaturationLimit1/1(SignalSatd) -> 0.2/1
  Drive_Signal1/5(OffsetOutput) -> Terminator5/1
  Amplitude/1 -> p2p to amp/1
  p2p to amp/1 -> Sum/1, Sum1/1
  Drive_Signal/4(AmplitudeOutput) -> Terminator3/1
  Drive_Signal1/2(WithoutRamp) -> Terminator6/1
  Drive_Signal1/3(RampOutput) -> Terminator7/1
  Drive_Signal1/4(AmplitudeOutput) -> Terminator9/1
  0.01/1 -> Bias_D2A/1
  0.1/1 -> D2A DriveSignal 1/1
  0.2/1 -> D2A DriveSignal 2/1
  Sum1/1 -> Drive_Signal1/4(Amplitude)
  Drive_Signal1/1(SignalOutput) -> SignalSaturationLimit1/2(SignalRaw)
  Drive_Signal/1(SignalOutput) -> SignalSaturationLimit/2(SignalRaw)
  Phase (deg)/1 -> Drive_Signal/6(Phase)
  Drive_Signal/6(WithoutRamp1) -> Terminator4/1
  PitchBias V (left)/1 -> Drive_Signal/5(PitchBias)
  a2/1 -> Drive_Signal/7("a2 "), Drive_Signal1/6(a2)
  PitchBias V (right)/1 -> Drive_Signal1/5(PitchBias)

== system target_driver_2022_Ctrl_v_2_4_landing_2017a/timer1 ==
  SaturatingRamp : DiscreteIntegrator  gainval=1  SampleTime=-1  UpperSaturationLimit=1  LowerSaturationLimit=0  ICPrevOutput=DiscIntNeverNeededParam  ICPrevScaledInput=DiscIntNeverNeededParam
  constant : Constant
  time : Outport
  wires:
  SaturatingRamp/1 -> time/1
  constant/1 -> SaturatingRamp/1
